simulink model "project"  (R2023b)
settings: Solver=FixedStepAuto  StartTime=0.0  StopTime=75  FixedStep=0.025  RelTol=1e-3
model workspace (MAT data in the model file):
  A : Simulink.Parameter (value not decoded)
  Aag : Simulink.Parameter (value not decoded)
  B : Simulink.Parameter (value not decoded)
  Bag : Simulink.Parameter (value not decoded)
  C : Simulink.Parameter (value not decoded)
  Cag : Simulink.Parameter (value not decoded)
  uang = [0 0 0 0 0 0 5.50670620214e-14 5.44009282066e-14 0 -3.99756362155e-05 -2.83106871279e-14 0 ... (9003 elements, 3x3001)]
  upos = [0 0 0 5.62466739851e-14 5.62327961973e-14 0 -2.39975660277e-05 4.94743135349e-14 0 -9.31686537426e-05 7.62168106405e-14 0 ... (9003 elements, 3x3001)]
libraries: neural x90, aerolibanimutils x1
(part 4 of 4)

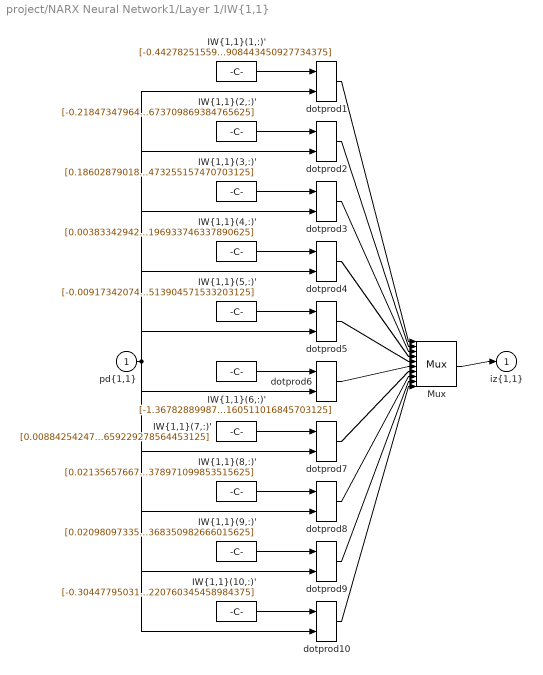
== system project/NARX Neural Network1/Layer 1/IW{1,1} ==
  "pd{1,1}" : Inport  PortDimensions=4  SampleTime=1
      mask Display: e = 0.06;c1 = [120 230 180]/255;c2 = ([120 230 180]+0)/(256+128);c3 = ([120 230 180]+128)/(256+128);patch([0 1 1 0],[0 0 1 1],c1);patch([0 1 1 1-e 1-e 0+e],[0 0 1 1-e 0+e 0+e],c2);patch([0 0 1 1-e 0+e 0+e],[0 1 1 1-e 1-e 0+e],c3);plot([0 1 1 0 0],[0 0 1 1 0]);
  "IW{1,1}(1,:)'" : Constant  Value=[-0.44278251559949233229218634733115322887897491455078125;1.2169181009199814269550188328139483928680419921875;-0.6925932951093038969503368207369931042194366455078125;0.8926953147872376259641669093980453908443450927734375]
      mask Display: e = 0.06;c1 = [120 150 230]/255;c2 = ([120 150 230]+0)/383;c3 = ([120 150 230]+128)/383;patch([0 1 1 0],[0 0 1 1],c1);patch([0 1 1 1-e 1-e 0+e],[0 0 1 1-e 0+e 0+e],c2);patch([0 0 1 1-e 0+e 0+e],[0 1 1 1-e 1-e 0+e],c3);plot([0 1 1 0 0],[0 0 1 1 0]);disp('Weights');
  "IW{1,1}(10,:)'" : Constant  Value=[-0.3044779503174037671442420105449855327606201171875;-0.0582249634909357827172726729259011335670948028564453125;0.250036232514247169778087709346436895430088043212890625;0.10019746822069862390858219214351265691220760345458984375]
      mask Display: e = 0.06;c1 = [120 150 230]/255;c2 = ([120 150 230]+0)/383;c3 = ([120 150 230]+128)/383;patch([0 1 1 0],[0 0 1 1],c1);patch([0 1 1 1-e 1-e 0+e],[0 0 1 1-e 0+e 0+e],c2);patch([0 0 1 1-e 0+e 0+e],[0 1 1 1-e 1-e 0+e],c3);plot([0 1 1 0 0],[0 0 1 1 0]);disp('Weights');
  "IW{1,1}(2,:)'" : Constant  Value=[-0.218473479645419466077527204106445424258708953857421875;0.483917986152067214344896228794823400676250457763671875;-0.5029090656065149378406431424082256853580474853515625;-1.2022881817054857922499877531663514673709869384765625]
      mask Display: e = 0.06;c1 = [120 150 230]/255;c2 = ([120 150 230]+0)/383;c3 = ([120 150 230]+128)/383;patch([0 1 1 0],[0 0 1 1],c1);patch([0 1 1 1-e 1-e 0+e],[0 0 1 1-e 0+e 0+e],c2);patch([0 0 1 1-e 0+e 0+e],[0 1 1 1-e 1-e 0+e],c3);plot([0 1 1 0 0],[0 0 1 1 0]);disp('Weights');
  "IW{1,1}(3,:)'" : Constant  Value=[0.1860287901821433553806173222255893051624298095703125;0.007159996300941507026138754810062891920097172260284423828125;-0.53158909978880963809189097446505911648273468017578125;-0.7712584573916754226985403875005431473255157470703125]
      mask Display: e = 0.06;c1 = [120 150 230]/255;c2 = ([120 150 230]+0)/383;c3 = ([120 150 230]+128)/383;patch([0 1 1 0],[0 0 1 1],c1);patch([0 1 1 1-e 1-e 0+e],[0 0 1 1-e 0+e 0+e],c2);patch([0 0 1 1-e 0+e 0+e],[0 1 1 1-e 1-e 0+e],c3);plot([0 1 1 0 0],[0 0 1 1 0]);disp('Weights');
  "IW{1,1}(4,:)'" : Constant  Value=[0.0038334294276004608585661781461340069654397666454315185546875;0.00061143203218667484429016401037415562313981354236602783203125;-0.004908291785235029298928299823501220089383423328399658203125;-0.000621200456531447440557125450055764304124750196933746337890625]
      mask Display: e = 0.06;c1 = [120 150 230]/255;c2 = ([120 150 230]+0)/383;c3 = ([120 150 230]+128)/383;patch([0 1 1 0],[0 0 1 1],c1);patch([0 1 1 1-e 1-e 0+e],[0 0 1 1-e 0+e 0+e],c2);patch([0 0 1 1-e 0+e 0+e],[0 1 1 1-e 1-e 0+e],c3);plot([0 1 1 0 0],[0 0 1 1 0]);disp('Weights');
  "IW{1,1}(5,:)'" : Constant  Value=[-0.00917342074784716597635192414372795610688626766204833984375;-0.003016657558930490277970815071739707491360604763031005859375;0.01145104900765258996997442153542579035274684429168701171875;0.00184399623320200965921611402364987952751107513904571533203125]
      mask Display: e = 0.06;c1 = [120 150 230]/255;c2 = ([120 150 230]+0)/383;c3 = ([120 150 230]+128)/383;patch([0 1 1 0],[0 0 1 1],c1);patch([0 1 1 1-e 1-e 0+e],[0 0 1 1-e 0+e 0+e],c2);patch([0 0 1 1-e 0+e 0+e],[0 1 1 1-e 1-e 0+e],c3);plot([0 1 1 0 0],[0 0 1 1 0]);disp('Weights');
  "IW{1,1}(6,:)'" : Constant  Value=[-1.3678288998794421171822932592476718127727508544921875;0.8239699212349200774241353428806178271770477294921875;1.0075331758833370177086408148170448839664459228515625;0.233947365989552846787802309336257167160511016845703125]
      mask Display: e = 0.06;c1 = [120 150 230]/255;c2 = ([120 150 230]+0)/383;c3 = ([120 150 230]+128)/383;patch([0 1 1 0],[0 0 1 1],c1);patch([0 1 1 1-e 1-e 0+e],[0 0 1 1-e 0+e 0+e],c2);patch([0 0 1 1-e 0+e 0+e],[0 1 1 1-e 1-e 0+e],c3);plot([0 1 1 0 0],[0 0 1 1 0]);disp('Weights');
  "IW{1,1}(7,:)'" : Constant  Value=[0.0088425424732701853047789342099349596537649631500244140625;0.001244726217410623177184181287202591192908585071563720703125;-0.0083364486805314434725300287709615076892077922821044921875;-0.000863107623943817838137182452129536613938398659229278564453125]
      mask Display: e = 0.06;c1 = [120 150 230]/255;c2 = ([120 150 230]+0)/383;c3 = ([120 150 230]+128)/383;patch([0 1 1 0],[0 0 1 1],c1);patch([0 1 1 1-e 1-e 0+e],[0 0 1 1-e 0+e 0+e],c2);patch([0 0 1 1-e 0+e 0+e],[0 1 1 1-e 1-e 0+e],c3);plot([0 1 1 0 0],[0 0 1 1 0]);disp('Weights');
  "IW{1,1}(8,:)'" : Constant  Value=[0.0213565766702875393934224490521955885924398899078369140625;0.002608624070742366317376959017337867408059537410736083984375;-0.0231470559533669649476816942978985025547444820404052734375;-0.0020708793045655683739969532553004682995378971099853515625]
      mask Display: e = 0.06;c1 = [120 150 230]/255;c2 = ([120 150 230]+0)/383;c3 = ([120 150 230]+128)/383;patch([0 1 1 0],[0 0 1 1],c1);patch([0 1 1 1-e 1-e 0+e],[0 0 1 1-e 0+e 0+e],c2);patch([0 0 1 1-e 0+e 0+e],[0 1 1 1-e 1-e 0+e],c3);plot([0 1 1 0 0],[0 0 1 1 0]);disp('Weights');
  "IW{1,1}(9,:)'" : Constant  Value=[0.0209809733597288890216692180956670199520885944366455078125;0.0028967734207828005864315823458809973089955747127532958984375;-0.02312217756139754720745571603401913307607173919677734375;-0.004339127219412313753166277052741861552931368350982666015625]
      mask Display: e = 0.06;c1 = [120 150 230]/255;c2 = ([120 150 230]+0)/383;c3 = ([120 150 230]+128)/383;patch([0 1 1 0],[0 0 1 1],c1);patch([0 1 1 1-e 1-e 0+e],[0 0 1 1-e 0+e 0+e],c2);patch([0 0 1 1-e 0+e 0+e],[0 1 1 1-e 1-e 0+e],c3);plot([0 1 1 0 0],[0 0 1 1 0]);disp('Weights');
  Mux : Mux  Inputs=10
      mask Display: e = 0.06;c1 = [120 150 230]/255;c2 = ([120 150 230]+0)/383;c3 = ([120 150 230]+128)/383;patch([0 1 1 0],[0 0 1 1],c1);patch([0 1 1 1-e 1-e 0+e],[0 0 1 1-e 0+e 0+e],c2);patch([0 0 1 1-e 0+e 0+e],[0 1 1 1-e 1-e 0+e],c3);plot([0 1 1 0 0],[0 0 1 1 0]);disp('Mux');
  dotprod{1..10} (10 alike) : neural/Weight Functions/dotprod
  "iz{1,1}" : Outport
      mask Display: e = 0.06;c1 = [120 230 180]/255;c2 = ([120 230 180]+0)/(256+128);c3 = ([120 230 180]+128)/(256+128);patch([0 1 1 0],[0 0 1 1],c1);patch([0 1 1 1-e 1-e 0+e],[0 0 1 1-e 0+e 0+e],c2);patch([0 0 1 1-e 0+e 0+e],[0 1 1 1-e 1-e 0+e],c3);plot([0 1 1 0 0],[0 0 1 1 0]);
  wires:
  "IW{1,1}(1,:)'"/1 -> dotprod1/1
  "pd{1,1}"/1 -> dotprod1/2, dotprod2/2, dotprod3/2, dotprod4/2, dotprod5/2, dotprod6/2, dotprod7/2, dotprod8/2, dotprod9/2, dotprod10/2
  dotprod1/1 -> Mux/1
  "IW{1,1}(2,:)'"/1 -> dotprod2/1
  dotprod2/1 -> Mux/2
  "IW{1,1}(3,:)'"/1 -> dotprod3/1
  dotprod3/1 -> Mux/3
  "IW{1,1}(4,:)'"/1 -> dotprod4/1
  dotprod4/1 -> Mux/4
  "IW{1,1}(5,:)'"/1 -> dotprod5/1
  dotprod5/1 -> Mux/5
  "IW{1,1}(6,:)'"/1 -> dotprod6/1
  dotprod6/1 -> Mux/6
  "IW{1,1}(7,:)'"/1 -> dotprod7/1
  dotprod7/1 -> Mux/7
  "IW{1,1}(8,:)'"/1 -> dotprod8/1
  dotprod8/1 -> Mux/8
  "IW{1,1}(9,:)'"/1 -> dotprod9/1
  dotprod9/1 -> Mux/9
  "IW{1,1}(10,:)'"/1 -> dotprod10/1
  dotprod10/1 -> Mux/10
  Mux/1 -> "iz{1,1}"/1

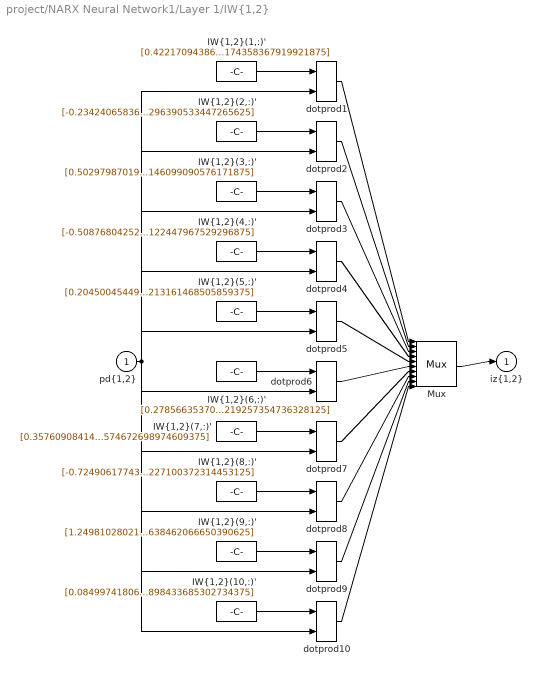
== system project/NARX Neural Network1/Layer 1/IW{1,2} ==
  "pd{1,2}" : Inport  PortDimensions=4  SampleTime=1
      mask Display: e = 0.06;c1 = [120 230 180]/255;c2 = ([120 230 180]+0)/(256+128);c3 = ([120 230 180]+128)/(256+128);patch([0 1 1 0],[0 0 1 1],c1);patch([0 1 1 1-e 1-e 0+e],[0 0 1 1-e 0+e 0+e],c2);patch([0 0 1 1-e 0+e 0+e],[0 1 1 1-e 1-e 0+e],c3);plot([0 1 1 0 0],[0 0 1 1 0]);
  "IW{1,2}(1,:)'" : Constant  Value=[0.42217094386850551046563850832171738147735595703125;-0.1520653883567786024411105927356402389705181121826171875;0.59689388854285929664200693878228776156902313232421875;-0.192719126234240867301394928290392272174358367919921875]
      mask Display: e = 0.06;c1 = [120 150 230]/255;c2 = ([120 150 230]+0)/383;c3 = ([120 150 230]+128)/383;patch([0 1 1 0],[0 0 1 1],c1);patch([0 1 1 1-e 1-e 0+e],[0 0 1 1-e 0+e 0+e],c2);patch([0 0 1 1-e 0+e 0+e],[0 1 1 1-e 1-e 0+e],c3);plot([0 1 1 0 0],[0 0 1 1 0]);disp('Weights');
  "IW{1,2}(10,:)'" : Constant  Value=[0.084997418061849294712573055221582762897014617919921875;-0.337208640053954289417248446625308133661746978759765625;-1.06060462981231307111329442705027759075164794921875;0.9889368639282645201404875479056499898433685302734375]
      mask Display: e = 0.06;c1 = [120 150 230]/255;c2 = ([120 150 230]+0)/383;c3 = ([120 150 230]+128)/383;patch([0 1 1 0],[0 0 1 1],c1);patch([0 1 1 1-e 1-e 0+e],[0 0 1 1-e 0+e 0+e],c2);patch([0 0 1 1-e 0+e 0+e],[0 1 1 1-e 1-e 0+e],c3);plot([0 1 1 0 0],[0 0 1 1 0]);disp('Weights');
  "IW{1,2}(2,:)'" : Constant  Value=[-0.23424065836421903430419888536562211811542510986328125;0.399966814621368349502716910137678496539592742919921875;0.57983048356221467134474778504227288067340850830078125;-0.09467114053461934963795698649846599437296390533447265625]
      mask Display: e = 0.06;c1 = [120 150 230]/255;c2 = ([120 150 230]+0)/383;c3 = ([120 150 230]+128)/383;patch([0 1 1 0],[0 0 1 1],c1);patch([0 1 1 1-e 1-e 0+e],[0 0 1 1-e 0+e 0+e],c2);patch([0 0 1 1-e 0+e 0+e],[0 1 1 1-e 1-e 0+e],c3);plot([0 1 1 0 0],[0 0 1 1 0]);disp('Weights');
  "IW{1,2}(3,:)'" : Constant  Value=[0.5029798701950056738496641628444194793701171875;-0.255843945989123522366526231053285300731658935546875;-0.344364597948892459111647212921525351703166961669921875;0.70818356173769714256849283628980629146099090576171875]
      mask Display: e = 0.06;c1 = [120 150 230]/255;c2 = ([120 150 230]+0)/383;c3 = ([120 150 230]+128)/383;patch([0 1 1 0],[0 0 1 1],c1);patch([0 1 1 1-e 1-e 0+e],[0 0 1 1-e 0+e 0+e],c2);patch([0 0 1 1-e 0+e 0+e],[0 1 1 1-e 1-e 0+e],c3);plot([0 1 1 0 0],[0 0 1 1 0]);disp('Weights');
  "IW{1,2}(4,:)'" : Constant  Value=[-0.5087680425238130244025569481891579926013946533203125;-0.464123858373629405438265393968322314321994781494140625;0.219379374547841787812529901202651672065258026123046875;0.152557991333091169661173580607282929122447967529296875]
      mask Display: e = 0.06;c1 = [120 150 230]/255;c2 = ([120 150 230]+0)/383;c3 = ([120 150 230]+128)/383;patch([0 1 1 0],[0 0 1 1],c1);patch([0 1 1 1-e 1-e 0+e],[0 0 1 1-e 0+e 0+e],c2);patch([0 0 1 1-e 0+e 0+e],[0 1 1 1-e 1-e 0+e],c3);plot([0 1 1 0 0],[0 0 1 1 0]);disp('Weights');
  "IW{1,2}(5,:)'" : Constant  Value=[0.2045004544950815572601499070515274070203304290771484375;-0.67366787613366174714002454493311233818531036376953125;0.1072878354840101911005234569529420696198940277099609375;0.440697398239986382062483016852638684213161468505859375]
      mask Display: e = 0.06;c1 = [120 150 230]/255;c2 = ([120 150 230]+0)/383;c3 = ([120 150 230]+128)/383;patch([0 1 1 0],[0 0 1 1],c1);patch([0 1 1 1-e 1-e 0+e],[0 0 1 1-e 0+e 0+e],c2);patch([0 0 1 1-e 0+e 0+e],[0 1 1 1-e 1-e 0+e],c3);plot([0 1 1 0 0],[0 0 1 1 0]);disp('Weights');
  "IW{1,2}(6,:)'" : Constant  Value=[0.278566353709527536608447917387820780277252197265625;0.29266535993370990098583206417970359325408935546875;0.0982406513600907194128097899010754190385341644287109375;-0.4550913367779572116234021450509317219257354736328125]
      mask Display: e = 0.06;c1 = [120 150 230]/255;c2 = ([120 150 230]+0)/383;c3 = ([120 150 230]+128)/383;patch([0 1 1 0],[0 0 1 1],c1);patch([0 1 1 1-e 1-e 0+e],[0 0 1 1-e 0+e 0+e],c2);patch([0 0 1 1-e 0+e 0+e],[0 1 1 1-e 1-e 0+e],c3);plot([0 1 1 0 0],[0 0 1 1 0]);disp('Weights');
  "IW{1,2}(7,:)'" : Constant  Value=[0.35760908414745584682492562933475710451602935791015625;0.83840959818871774178461464543943293392658233642578125;-0.06231099879840680533238383986827102489769458770751953125;-0.518237682005382449546004863805137574672698974609375]
      mask Display: e = 0.06;c1 = [120 150 230]/255;c2 = ([120 150 230]+0)/383;c3 = ([120 150 230]+128)/383;patch([0 1 1 0],[0 0 1 1],c1);patch([0 1 1 1-e 1-e 0+e],[0 0 1 1-e 0+e 0+e],c2);patch([0 0 1 1-e 0+e 0+e],[0 1 1 1-e 1-e 0+e],c3);plot([0 1 1 0 0],[0 0 1 1 0]);disp('Weights');
  "IW{1,2}(8,:)'" : Constant  Value=[-0.7249061774370415545121204559109173715114593505859375;-0.135570236626455675743585516102029941976070404052734375;0.424848466168581906376999768326641060411930084228515625;-0.18973629321811291692512213558075018227100372314453125]
      mask Display: e = 0.06;c1 = [120 150 230]/255;c2 = ([120 150 230]+0)/383;c3 = ([120 150 230]+128)/383;patch([0 1 1 0],[0 0 1 1],c1);patch([0 1 1 1-e 1-e 0+e],[0 0 1 1-e 0+e 0+e],c2);patch([0 0 1 1-e 0+e 0+e],[0 1 1 1-e 1-e 0+e],c3);plot([0 1 1 0 0],[0 0 1 1 0]);disp('Weights');
  "IW{1,2}(9,:)'" : Constant  Value=[1.2498102802148698398099213591194711625576019287109375;0.100982913778056959674955805894569493830204010009765625;-0.9862271682086267698963411021395586431026458740234375;-0.2850756182866513999130120282643474638462066650390625]
      mask Display: e = 0.06;c1 = [120 150 230]/255;c2 = ([120 150 230]+0)/383;c3 = ([120 150 230]+128)/383;patch([0 1 1 0],[0 0 1 1],c1);patch([0 1 1 1-e 1-e 0+e],[0 0 1 1-e 0+e 0+e],c2);patch([0 0 1 1-e 0+e 0+e],[0 1 1 1-e 1-e 0+e],c3);plot([0 1 1 0 0],[0 0 1 1 0]);disp('Weights');
  Mux : Mux  Inputs=10
      mask Display: e = 0.06;c1 = [120 150 230]/255;c2 = ([120 150 230]+0)/383;c3 = ([120 150 230]+128)/383;patch([0 1 1 0],[0 0 1 1],c1);patch([0 1 1 1-e 1-e 0+e],[0 0 1 1-e 0+e 0+e],c2);patch([0 0 1 1-e 0+e 0+e],[0 1 1 1-e 1-e 0+e],c3);plot([0 1 1 0 0],[0 0 1 1 0]);disp('Mux');
  dotprod{1..10} (10 alike) : neural/Weight Functions/dotprod
  "iz{1,2}" : Outport
      mask Display: e = 0.06;c1 = [120 230 180]/255;c2 = ([120 230 180]+0)/(256+128);c3 = ([120 230 180]+128)/(256+128);patch([0 1 1 0],[0 0 1 1],c1);patch([0 1 1 1-e 1-e 0+e],[0 0 1 1-e 0+e 0+e],c2);patch([0 0 1 1-e 0+e 0+e],[0 1 1 1-e 1-e 0+e],c3);plot([0 1 1 0 0],[0 0 1 1 0]);
  wires:
  "IW{1,2}(1,:)'"/1 -> dotprod1/1
  "pd{1,2}"/1 -> dotprod1/2, dotprod2/2, dotprod3/2, dotprod4/2, dotprod5/2, dotprod6/2, dotprod7/2, dotprod8/2, dotprod9/2, dotprod10/2
  dotprod1/1 -> Mux/1
  "IW{1,2}(2,:)'"/1 -> dotprod2/1
  dotprod2/1 -> Mux/2
  "IW{1,2}(3,:)'"/1 -> dotprod3/1
  dotprod3/1 -> Mux/3
  "IW{1,2}(4,:)'"/1 -> dotprod4/1
  dotprod4/1 -> Mux/4
  "IW{1,2}(5,:)'"/1 -> dotprod5/1
  dotprod5/1 -> Mux/5
  "IW{1,2}(6,:)'"/1 -> dotprod6/1
  dotprod6/1 -> Mux/6
  "IW{1,2}(7,:)'"/1 -> dotprod7/1
  dotprod7/1 -> Mux/7
  "IW{1,2}(8,:)'"/1 -> dotprod8/1
  dotprod8/1 -> Mux/8
  "IW{1,2}(9,:)'"/1 -> dotprod9/1
  dotprod9/1 -> Mux/9
  "IW{1,2}(10,:)'"/1 -> dotprod10/1
  dotprod10/1 -> Mux/10
  Mux/1 -> "iz{1,2}"/1

== system project/NARX Neural Network1/Layer 2/Delays 1 ==
  "p{2}" : Inport  PortDimensions=10  SampleTime=1
      mask Display: e = 0.06;c1 = [120 230 180]/255;c2 = ([120 230 180]+0)/(256+128);c3 = ([120 230 180]+128)/(256+128);patch([0 1 1 0],[0 0 1 1],c1);patch([0 1 1 1-e 1-e 0+e],[0 0 1 1-e 0+e 0+e],c2);patch([0 0 1 1-e 0+e 0+e],[0 1 1 1-e 1-e 0+e],c3);plot([0 1 1 0 0],[0 0 1 1 0]);
  mux : Mux  Inputs=1
      mask Display: e = 0.06;c1 = [120 150 230]/255;c2 = ([120 150 230]+0)/383;c3 = ([120 150 230]+128)/383;patch([0 1 1 0],[0 0 1 1],c1);patch([0 1 1 1-e 1-e 0+e],[0 0 1 1-e 0+e 0+e],c2);patch([0 0 1 1-e 0+e 0+e],[0 1 1 1-e 1-e 0+e],c3);plot([0 1 1 0 0],[0 0 1 1 0]);disp('Mux')
  "pd{2,1}" : Outport
      mask Display: e = 0.06;c1 = [120 230 180]/255;c2 = ([120 230 180]+0)/(256+128);c3 = ([120 230 180]+128)/(256+128);patch([0 1 1 0],[0 0 1 1],c1);patch([0 1 1 1-e 1-e 0+e],[0 0 1 1-e 0+e 0+e],c2);patch([0 0 1 1-e 0+e 0+e],[0 1 1 1-e 1-e 0+e],c3);plot([0 1 1 0 0],[0 0 1 1 0]);
  wires:
  "p{2}"/1 -> mux/1
  mux/1 -> "pd{2,1}"/1

== system project/NARX Neural Network1/Layer 2/LW{2,1} ==
  "ad{2,1}" : Inport  PortDimensions=10  SampleTime=1
      mask Display: e = 0.06;c1 = [120 230 180]/255;c2 = ([120 230 180]+0)/(256+128);c3 = ([120 230 180]+128)/(256+128);patch([0 1 1 0],[0 0 1 1],c1);patch([0 1 1 1-e 1-e 0+e],[0 0 1 1-e 0+e 0+e],c2);patch([0 0 1 1-e 0+e 0+e],[0 1 1 1-e 1-e 0+e],c3);plot([0 1 1 0 0],[0 0 1 1 0]);
  "IW{2,1}(1,:)'" : Constant  Value=[0.0010261702296776413489975965376288513652980327606201171875;-0.0003078558682555836947987437657303644300554879009723663330078125;-0.000620152438584861578733942177876770074362866580486297607421875;-1.0225307087195847355332034567254595458507537841796875;1.2506159953489144331939542098552919924259185791015625;0.002303874945676507614289452163802707218565046787261962890625;0.638300824792421561681976527324877679347991943359375;-0.98058164226623978354524524547741748392581939697265625;0.87091374708742741450606672515277750790119171142578125;-0.218336024350647084357746052774018608033657073974609375]
      mask Display: e = 0.06;c1 = [120 150 230]/255;c2 = ([120 150 230]+0)/383;c3 = ([120 150 230]+128)/383;patch([0 1 1 0],[0 0 1 1],c1);patch([0 1 1 1-e 1-e 0+e],[0 0 1 1-e 0+e 0+e],c2);patch([0 0 1 1-e 0+e 0+e],[0 1 1 1-e 1-e 0+e],c3);plot([0 1 1 0 0],[0 0 1 1 0]);disp('weights');
  "IW{2,1}(2,:)'" : Constant  Value=[9.020315386256915987130133860461000949726440012454986572265625e-05;-0.00061034417662448291197474503633202402852475643157958984375;-0.0006985074788832036120356239194961744942702353000640869140625;-1.38025675783678902774909147410653531551361083984375;-1.3626056442823462067082118664984591305255889892578125;-0.0002718109136974126397064133175973665856872685253620147705078125;0.90048385257446128537850427164812572300434112548828125;-1.2645666958503458676688069317606277763843536376953125;-0.54865007039056890025818802314461208879947662353515625;0.0967570550481110236429316273643053136765956878662109375]
      mask Display: e = 0.06;c1 = [120 150 230]/255;c2 = ([120 150 230]+0)/383;c3 = ([120 150 230]+128)/383;patch([0 1 1 0],[0 0 1 1],c1);patch([0 1 1 1-e 1-e 0+e],[0 0 1 1-e 0+e 0+e],c2);patch([0 0 1 1-e 0+e 0+e],[0 1 1 1-e 1-e 0+e],c3);plot([0 1 1 0 0],[0 0 1 1 0]);disp('weights');
  Mux : Mux  Inputs=2
      mask Display: e = 0.06;c1 = [120 150 230]/255;c2 = ([120 150 230]+0)/383;c3 = ([120 150 230]+128)/383;patch([0 1 1 0],[0 0 1 1],c1);patch([0 1 1 1-e 1-e 0+e],[0 0 1 1-e 0+e 0+e],c2);patch([0 0 1 1-e 0+e 0+e],[0 1 1 1-e 1-e 0+e],c3);plot([0 1 1 0 0],[0 0 1 1 0]);disp('Mux');
  dotprod1 : neural/Weight Functions/dotprod
  dotprod2 : neural/Weight Functions/dotprod
  "lz{2,1}" : Outport
      mask Display: e = 0.06;c1 = [120 230 180]/255;c2 = ([120 230 180]+0)/(256+128);c3 = ([120 230 180]+128)/(256+128);patch([0 1 1 0],[0 0 1 1],c1);patch([0 1 1 1-e 1-e 0+e],[0 0 1 1-e 0+e 0+e],c2);patch([0 0 1 1-e 0+e 0+e],[0 1 1 1-e 1-e 0+e],c3);plot([0 1 1 0 0],[0 0 1 1 0]);
  wires:
  "IW{2,1}(1,:)'"/1 -> dotprod1/1
  "ad{2,1}"/1 -> dotprod1/2, dotprod2/2
  dotprod1/1 -> Mux/1
  "IW{2,1}(2,:)'"/1 -> dotprod2/1
  dotprod2/1 -> Mux/2
  Mux/1 -> "lz{2,1}"/1

== matlab function project/Quadrotor Dynamics/MATLAB Function8 ==
  data: ball output; ypos input; lr input; ls input
function ball= balll(ypos,lr,ls)
ball=[ypos(1)+lr(1) -(ypos(2)+ls(1)) 1-ypos(3)-sqrt(0.25-lr(1)^2-ls(1)^2)]';

== matlab function project/MATLAB Function ==
  data: upos input; y output; t input
function y = fcn(upos,t)
T = floor(t/0.025)+1;
y = upos(:,T);

== matlab function project/MATLAB Function4 ==
  data: uang input; y output; t input
function y= fcn(uang,t)
T = floor(t/0.025)+1;
y = uang(:,T);

== matlab function project/Quadrotor Dynamics/MATLAB Function2 ==
  data: yang output; xang output; u input; xangi input
function [yang,xang]= sysang(u,xangi)
Ts = 1/40;
g = 9.81;
A = [1,0.0250000000000000,0,0,0,0;0,1,0,0,0,0;0,0,1,0.0250000000000000,0,0;0,0,0,1,0,0;0,0,0,0,1,0.0250000000000000;0,0,0,0,0,1];
B = [0.0416666666666667,0,0;3.33333333333333,0,0;0,0.0416666666666667,0;0,3.33333333333333,0;0,0,0.0240384615384615;0,0,1.92307692307692];
C = [1,0,0,0,0,0;0,0,1,0,0,0;0,0,0,0,1,0];
D = zeros(3,3);
xang = A*xangi + B*u;
yang = C*xang + D*u;

== matlab function project/Quadrotor Dynamics/MATLAB Function3 ==
  data: y output; x output; u input; xi input; fx input; fy input; fx output; fy output; ls input; lr input; ls output; lr output; vr input; vs input; vr output; vs output; sdold input; sdold output
function [y,x, fx,fy,ls,lr,vr,vs,sdold]= syspos(u,xi,fx,fy,ls,lr,vr,vs,sdold)
Ts = 1/40;
g = 9.81;
A = [1 0.025 0 0 0 0;0 1 0 0 0 0;0 0 1 0.025 0 0;0 0 0 1 0 0;0 0 0 0 1 0.025;0 0 0 0 0 1];
B = [-0.003065625 0 0;-0.24525 0 0;0 0.003065625 0;0 0.24525 0;0 0 0.0003125;0 0 0.025];
C = [1 0 0 0 0 0;0 0 1 0 0 0;0 0 0 0 1 0];
D = zeros(3,3);
x = A*xi + B*u;
y = C*x + D*u;
x(2) = x(2) - fx;
x(4) = x(4) - fy;


xdold = x(2)-xi(2);
ydold = x(4)-xi(4);
zdold = x(6)-xi(6);

yita = sqrt(0.5^2-lr^2-ls^2);
vrold = vr;
vsold = vs;
vr = ( yita^4*xdold - lr*yita^3*zdold + lr*ls*yita^2*sdold +...
    (lr*0.5^2-lr*ls^2)*vr^2 +...
    (lr*0.5^2-lr^3)*vs^2 +...
    2*vr*vs*lr^2*ls + lr*g*yita^3 )/((ls^2-0.5^2)*yita^2);
lr = lr + vr*Ts;
rdold = vr-vrold;

vs = ( yita^4*ydold - ls*yita^3*zdold + lr*ls*yita^2*rdold +...
    (ls*0.5^2-ls*lr^2)*vs^2 +...
    (ls*0.5^2-ls^3)*vr^2 +...
    2*vr*vs*ls^2*lr + ls*g*yita^3 )/((lr^2-0.5^2)*yita^2);
ls = ls + vs*Ts;
% sdold = vs(1,i+1);
sdold = vs(1)-vsold(1);

fx = 0.3*(xdold+rdold);
fy = 0.3*(ydold+sdold);

== matlab function project/Quadrotor Dynamics/MATLAB Function5 ==
  data: t input; u input; s input; plot input; enable input; ball input
function qd_plot(t,u,s, plot, enable,ball)
    quad.nrotors =4;
    quad.d = 0.17;
    quad.r = 0.1;
    
    a1s = zeros(1, quad.nrotors);
    b1s = zeros(1, quad.nrotors);

    
    % vehicle dimensons
    d = quad.d; %Hub displacement from COG
    r = quad.r; %Rotor radius
    D = zeros(3,4);
    C = zeros(3,4);
    for i = 1:quad.nrotors
        theta = (i-1)/quad.nrotors*2*pi;
        %   Di      Rotor hub displacements (1x3)
        % first rotor is on the x-axis, clockwise order looking down from above
        D(:,i) = [ d*cos(theta); d*sin(theta); 0];
%         scal = s(1)/4;
        scal = 0.2/4;
        %Attitude center displacements
        C(:,i) = [ scal*cos(theta); scal*sin(theta); 0];
    end
    
    if enable == 1
        %draw ground
        figure(plot);
        clf;
        if length(s) == 1
            axis([-0.5 1.5 -0.5 1.5 0 2]);
        else
%             axis([-s(1) s(1) -s(1) s(1) 0 s(2)])
            axis([-0.5 s(1) -0.5 s(1) 0 s(2)])
            s = 1.5;
        end
        hold on;
        
        % plot the ground boundaries and the big cross
        plot3([-0.5 -0.5],[-0.5 1],[0 0],'-b')
        plot3([-0.5 1.5],[-0.5 -0.5],[0 0],'-b')
        plot3([-0.5 1.5],[-0.5 1.5],[0 0],'-b')
        plot3([1.5 -0.5],[1.5 1.5],[0 0],'-b')
        plot3([1.5 1.5],[1.5 -0.5],[0 0],'-b')
        plot3([-0.5 1.5],[1.5 -0.5],[0 0],'-b')
        
        plot3([0 1], [0 0], [1.5 1.5],':r','LineWidth',0.2)
        plot3([1 1], [0 1], [1.5 1.5],':r','LineWidth',0.2)
        plot3([0 1], [1 1], [1.5 1.5],':r','LineWidth',0.2)
        plot3([0 0], [0 1], [1.5 1.5],':r','LineWidth',0.2)
        
        plot3([0 1], [0 0], [1 1],':r','LineWidth',0.2)
        plot3([1 1], [0 1], [1 1],':r','LineWidth',0.2)
        plot3([0 1], [1 1], [1 1],':r','LineWidth',0.2)
        plot3([0 0], [0 1], [1 1],':r','LineWidth',0.2)
        %READ STATE
        z = [u(1);u(2);u(3)];
        n = [u(4);u(5);u(6)];
        
        %PREPROCESS ROTATION MATRIX
        phi = n(1);    %Euler angles
        the = n(2);
        psi = n(3);
        
        R = [cos(the)*cos(phi) sin(psi)*sin(the)*cos(phi)-cos(psi)*sin(phi) cos(psi)*sin(the)*cos(phi)+sin(psi)*sin(phi);   %BBF > Inertial rotation matrix
            cos(the)*sin(phi) sin(psi)*sin(the)*sin(phi)+cos(psi)*cos(phi) cos(psi)*sin(the)*sin(phi)-sin(psi)*cos(phi);
            -sin(the)         sin(psi)*cos(the)                            cos(psi)*cos(the)];
        
        %Manual Construction
        %Q3 = [cos(psi) -sin(psi) 0;sin(psi) cos(psi) 0;0 0 1];   %Rotation mappings
        %Q2 = [cos(the) 0 sin(the);0 1 0;-sin(the) 0 cos(the)];
        %Q1 = [1 0 0;0 cos(phi) -sin(phi);0 sin(phi) cos(phi)];
        %R = Q3*Q2*Q1;    %Rotation matrix
        
        %CALCULATE FLYER TIP POSITONS USING COORDINATE FRAME ROTATION
        F = [1 0 0;0 -1 0;0 0 -1];
        
        %Draw flyer rotors
        t = [0:pi/8:2*pi];
        circle = zeros(3,17);
        for j = 1:length(t)
            circle(:,j) = [r*sin(t(j));r*cos(t(j));0];
        end
        hub = zeros(3,4);
        tippath = zeros(3,17,4);
        for i = 1:quad.nrotors
            hub(:,i) = F*(z + R*D(:,i)); %points in the inertial frame
            center = F*z;
            ball_pos = F*ball;
            plot3(center(1),center(2),center(3),'r.')
            plot3(ball_pos(1),ball_pos(2),ball_pos(3),'co')
            plot3([center(1) ball_pos(1)],[center(2) ball_pos(2)],[center(3) ball_pos(3)],'-b')
            
            q = 1; %Flapping angle scaling for output display - makes it easier to see what flapping is occurring
            Rr = [cos(q*a1s(i))  sin(q*b1s(i))*sin(q*a1s(i)) cos(q*b1s(i))*sin(q*a1s(i));   %Rotor > Plot frame
                0              cos(q*b1s(i))               -sin(q*b1s(i));
                -sin(q*a1s(i)) sin(q*b1s(i))*cos(q*a1s(i)) cos(q*b1s(i))*cos(q*a1s(i))];
            
            tippath(:,:,i) = F*R*Rr*circle;
            plot3([hub(1,i)+tippath(1,:,i)],[hub(2,i)+tippath(2,:,i)],[hub(3,i)+tippath(3,:,i)],'b-')
        end
        
        %Draw flyer
        hub0 = F*z;  % centre of vehicle
        for i = 1:quad.nrotors
            % line from hub to centre plot3([hub(1,N) hub(1,S)],[hub(2,N) hub(2,S)],[hub(3,N) hub(3,S)],'-b')
            plot3([hub(1,i) hub0(1)],[hub(2,i) hub0(2)],[hub(3,i) hub0(3)],'-b')
            
            % plot a circle at the hub itself
            plot3([hub(1,i)],[hub(2,i)],[hub(3,i)],'o')
        end
        
        % plot the vehicle's centroid on the ground plane
        plot3([z(1) 0],[-z(2) 0],[0 0],'--k')
        plot3([z(1)],[-z(2)],[0],'xk')
        plot3([z(1) z(1)],[-z(2) -s],[0 0],'r-.')

        % label the axes
        xlabel('x');
        ylabel('y');
        zlabel('z (height above ground)');
        view([-5 -2 5]);
    end;

== matlab function project/Quadrotor Dynamics/MATLAB Function6 ==
  data: up output; ypos input; yang input
function up= upp(ypos,yang)
up = [ypos(1) -ypos(2) -ypos(3) yang(1) yang(2) yang(3)];
